simulink model "RotationMotorSimulink"  (R2020b)
settings: Solver=VariableStepAuto  StartTime=0.0  StopTime=SimTime  RelTol=1e-3
InitFcn:
  | StartupScript
  | 
StartFcn:
  | StartupScript
values from neighbouring files (symbols this model uses):
  CF = 372.0    (= 372)    [StartupScript.m]
  GearRatior = 2.0    (= 2)    [StartupScript.m]
  Isat = 10.0    (= 10)    [StartupScript.m]
  Kdr = 3.4    [StartupScript.m]
  Kir = 6.1    [StartupScript.m]
  Kmr = 29.9*1e-3    (= 0.0299)    [StartupScript.m]
  Kpr = 40    [StartupScript.m]
  Kr = 1    [StartupScript.m]
  PidLim = 1024    [StartupScript.m]
  PidUCGain = 5/1024    (= 0.0048828125)    [StartupScript.m]
  r2d = 180/pi    (= 57.2957795131)    [StartupScript.m]
  sensorGain = 1/1024.0    (= 0.0009765625)    [StartupScript.m]
  Vsat = 24.0    (= 24)    [StartupScript.m]
libraries: cstblocks x4
settings Model: Creator=nisch  LastModifiedBy=miyaz

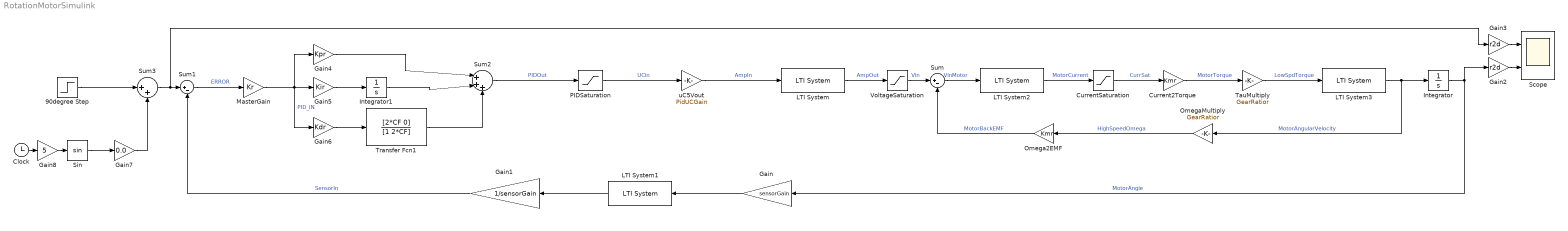
== system RotationMotorSimulink ==
  90degree Step : Step  Time=0  After=pi  SampleTime=0
  Clock : Clock
  Current2Torque : Gain  Gain=Kmr
  CurrentSaturation : Saturate  UpperLimit=Isat  LowerLimit=-Isat
  Gain : Gain  Gain=sensorGain
  Gain1 : Gain  Gain=1/sensorGain
  Gain2 : Gain  Gain=r2d
  Gain3 : Gain  Gain=r2d
  Gain4 : Gain  Gain=Kpr
  Gain5 : Gain  Gain=Kir
  Gain6 : Gain  Gain=Kdr
  Gain7 : Gain  Gain=0.0
  Gain8 : Gain  Gain=5
  Integrator : Integrator
  Integrator1 : Integrator
  LTI System : cstblocks/LTI System  sys=VoltageAmplifier  IC=[]
  LTI System1 : cstblocks/LTI System  sys=Hs  IC=[]
  LTI System2 : cstblocks/LTI System  sys=Electricalr  IC=[]
  LTI System3 : cstblocks/LTI System  sys=Mechanicalr  IC=[]
  MasterGain : Gain  Gain=Kr
  Omega2EMF : Gain  Gain=Kmr
  OmegaMultiply : Gain  Gain=GearRatior
  PIDSaturation : Saturate  UpperLimit=PidLim  LowerLimit=-PidLim
  Scope : Scope  NumInputPorts=2
  Sin : Trigonometry
  Sum : Sum  Inputs=|+-
  Sum1 : Sum  Inputs=|+-
  Sum2 : Sum  Inputs=|+++
  Sum3 : Sum  Inputs=|++
  TauMultiply : Gain  Gain=GearRatior
  Transfer Fcn1 : TransferFcn  Numerator=[2*CF 0]  Denominator=[1 2*CF]
  VoltageSaturation : Saturate  UpperLimit=Vsat  LowerLimit=-Vsat
  uC5Vout : Gain  Gain=PidUCGain
  wires:
  Gain7/1 -> Sum3/2
  LTI System/1 -> VoltageSaturation/1  "AmpOut"
  PIDSaturation/1 -> uC5Vout/1  "UCin"
  Sin/1 -> Gain7/1
  Gain8/1 -> Sin/1
  VoltageSaturation/1 -> Sum/1  "Vin"
  Sum3/1 -> Gain3/1, Sum1/1
  uC5Vout/1 -> LTI System/1  "AmpIn"
  Current2Torque/1 -> TauMultiply/1  "MotorTorque"
  TauMultiply/1 -> LTI System3/1  "LowSpdTorque"
  Gain/1 -> LTI System1/1
  OmegaMultiply/1 -> Omega2EMF/1  "HighSpeedOmega"
  Gain6/1 -> Transfer Fcn1/1
  Gain5/1 -> Integrator1/1
  Sum1/1 -> MasterGain/1  "ERROR"
  LTI System2/1 -> CurrentSaturation/1  "MotorCurrent"
  CurrentSaturation/1 -> Current2Torque/1  "CurrSat"
  Integrator/1 -> Gain2/1, Gain/1  "MotorAngle"
  LTI System3/1 -> Integrator/1, OmegaMultiply/1  "MotorAngularVelocity"
  Gain2/1 -> Scope/2
  90degree Step/1 -> Sum3/1
  Clock/1 -> Gain8/1
  Transfer Fcn1/1 -> Sum2/3
  Sum/1 -> LTI System2/1  "VinMotor"
  Gain4/1 -> Sum2/1
  Integrator1/1 -> Sum2/2
  MasterGain/1 -> Gain6/1, Gain5/1, Gain4/1  "PID_IN"
  Sum2/1 -> PIDSaturation/1  "PIDOut"
  Omega2EMF/1 -> Sum/2  "MotorBackEMF"
  LTI System1/1 -> Gain1/1
  Gain1/1 -> Sum1/2  "SensorIn"
  Gain3/1 -> Scope/1
